simulink model "IDCS_nonlinear"  (R2018a)
settings: Solver=ode4  StartTime=0.0  StopTime=t_end  FixedStep=Step_Time  RelTol=1e-3
values from neighbouring files (symbols this model uses):
  A = [ 0 0 1 0 ... (first row only)    [bode_IDCS.m]    (also in bode_hiratsuka_IDCS.m = 1; hiratsuka_IDCS.m = 0.003; model_IDCS.m = 0.003; model_hiratsuka_nondamper.m = 0.003)
  Aor = 0.1*10^-6    (= 1e-07)    [bode_hiratsuka_IDCS.m]    (also in hiratsuka_IDCS.m; model_hiratsuka_nondamper.m; model_nonlinear_damper.m; model_nonlinear_nondamper.m)
  Ap = (32.50*0.001)^2*pi/4    (= 0.000829576810089)    [bode_hiratsuka_IDCS.m]    (also in hiratsuka_IDCS.m; model_hiratsuka_nondamper.m; model_nonlinear_damper.m; model_nonlinear_nondamper.m)
  B = [0; 0; k1/m1; 0]    [bode_IDCS.m]    (also in bode_hiratsuka_IDCS.m = 0; hiratsuka_IDCS.m = 0; model_hiratsuka_nondamper.m = 0; model_nonlinear_damper.m = 0)
  c1 = 150    [bode_hiratsuka_IDCS.m]    (also in hiratsuka_IDCS.m = 5; model_IDCS.m = 5; model_hiratsuka_nondamper.m = 15; model_linear_damper.m = 50)
  c2 = 7    [bode_IDCS.m]    (also in bode_hiratsuka_IDCS.m; hiratsuka_IDCS.m; model_IDCS.m; model_hiratsuka_nondamper.m)
  Cor = 0.8    [bode_hiratsuka_IDCS.m]    (also in hiratsuka_IDCS.m; model_hiratsuka_nondamper.m; model_nonlinear_damper.m; model_nonlinear_nondamper.m)
  Hz = wv(k)    [bode_hiratsuka_IDCS.m]    (also in hiratsuka_IDCS.m = 6.28318530718; model_IDCS.m = 6.28318530718; model_hiratsuka_nondamper.m = 6.28318530718; model_linear_damper.m = 18.8495559215)
  k1 = 2200    [bode_IDCS.m]    (also in bode_hiratsuka_IDCS.m; hiratsuka_IDCS.m; model_IDCS.m; model_hiratsuka_nondamper.m)
  k2 = 405    [bode_IDCS.m]    (also in bode_hiratsuka_IDCS.m; hiratsuka_IDCS.m; model_IDCS.m; model_hiratsuka_nondamper.m)
  kappa = 1.4    [bode_hiratsuka_IDCS.m]    (also in hiratsuka_IDCS.m; model_hiratsuka_nondamper.m; model_nonlinear_damper.m; model_nonlinear_nondamper.m)
  Kp = 500    [bode_IDCS.m]    (also in bode_hiratsuka_IDCS.m = 80; hiratsuka_IDCS.m = 60; model_IDCS.m = 100; model_hiratsuka_nondamper.m = 80)
  m1 = 1.5    [bode_IDCS.m]    (also in bode_hiratsuka_IDCS.m; hiratsuka_IDCS.m; model_IDCS.m; model_hiratsuka_nondamper.m)
  m2 = 6.4    [bode_IDCS.m]    (also in bode_hiratsuka_IDCS.m; hiratsuka_IDCS.m; model_IDCS.m; model_hiratsuka_nondamper.m)
  P0 = 101325    [bode_hiratsuka_IDCS.m]    (also in hiratsuka_IDCS.m; model_hiratsuka_nondamper.m; model_nonlinear_damper.m; model_nonlinear_nondamper.m)
  row0 = 1.1841    [bode_hiratsuka_IDCS.m]    (also in hiratsuka_IDCS.m; model_hiratsuka_nondamper.m; model_nonlinear_damper.m; model_nonlinear_nondamper.m)
  T_diff = 1/(2*pi*cutoff)    (= 0.00795774715459)    [bode_IDCS.m]    (also in hiratsuka_IDCS.m = 0.00159154943092; model_IDCS.m = 0.00159154943092; model_hiratsuka_nondamper.m = 0.00159154943092; model_linear_damper.m)
  x0 = 0.05    [bode_hiratsuka_IDCS.m]    (also in hiratsuka_IDCS.m = 0.042; model_hiratsuka_nondamper.m; model_nonlinear_damper.m = 0.042; model_nonlinear_nondamper.m = 0.042)
undefined symbols (not defined in the file or in its folder): Kd, Ki
libraries: simulink x1
settings Model: Creator=Natsu Nakagawa  LastModifiedBy=Natsu Nakagawa
settings DataIOCC: ReturnWorkspaceOutputs=on
settings SFSimCC: SimUseLocalCustomCode=on
settings RTWCC: RTWUseLocalCustomCode=on

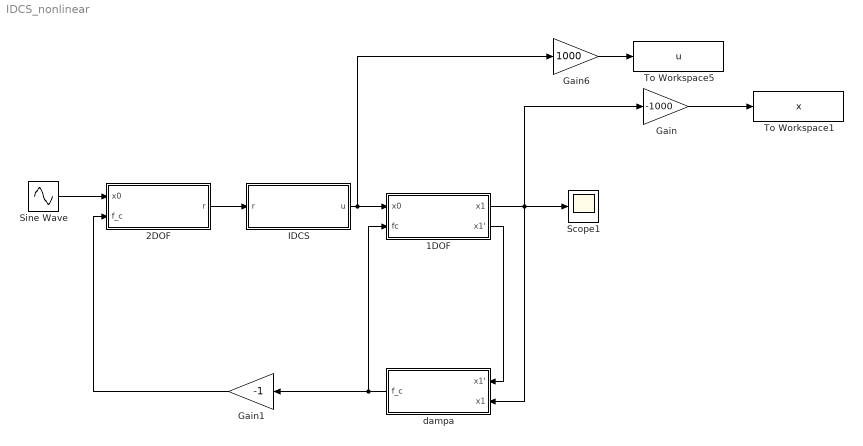
== system IDCS_nonlinear ==
  1DOF : Subsystem
  2DOF : Subsystem
  Gain : Gain  Gain=-1000
  Gain1 : Gain  Gain=-1
  Gain6 : Gain  Gain=1000
  IDCS : Subsystem
  Scope1 : Scope
  Sine Wave : Sin  Amplitude=A  Bias=B  Frequency=Hz  SampleTime=0
  To Workspace1 : ToWorkspace  VariableName=x  SaveFormat=Timeseries  SampleTime=-1
  To Workspace5 : ToWorkspace  VariableName=u  SaveFormat=Timeseries  SampleTime=-1
  dampa : Subsystem
  wires:
  1DOF/1(x1) -> Gain/1, dampa/2(x1), Scope1/1
  2DOF/1(r) -> IDCS/1(r)
  Sine Wave/1 -> 2DOF/1(x0)
  Gain6/1 -> To Workspace5/1
  Gain/1 -> To Workspace1/1
  IDCS/1(u) -> Gain6/1, 1DOF/1(x0)
  1DOF/2(x1') -> dampa/1(x1')
  dampa/1(f_c) -> Gain1/1, 1DOF/2(fc)
  Gain1/1 -> 2DOF/2(f_c)

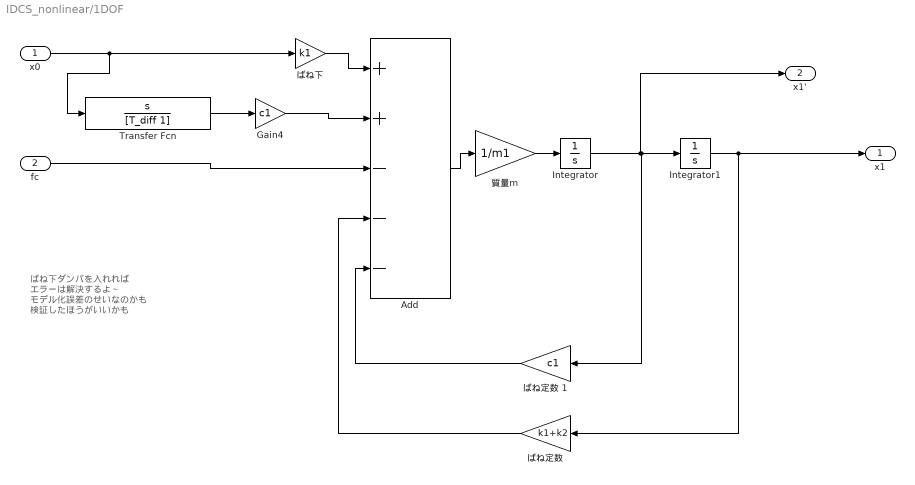
== system IDCS_nonlinear/1DOF ==
  note: ばね下ダンパを入れれば
      | エラーは解決するよ～
      | モデル化誤差のせいなのかも
      | 検証したほうがいいかも
  x0 : Inport
  fc : Inport  Port=2
  Add : Sum  Inputs=++---
  Gain4 : Gain  Gain=c1
  Integrator : Integrator
  Integrator1 : Integrator
  Transfer Fcn : TransferFcn  Numerator=[1, 0]  Denominator=[T_diff 1]
  ばね下 : Gain  Gain=k1
  "ばね定数 " : Gain  Gain=k1+k2
  ばね定数 1 : Gain  Gain=c1
  質量m : Gain  Gain=1/m1
  x1 : Outport
  x1' : Outport  Port=2
  wires:
  Integrator/1 -> x1'/1, ばね定数 1/1, Integrator1/1
  Add/1 -> 質量m/1
  質量m/1 -> Integrator/1
  Integrator1/1 -> x1/1, "ばね定数 "/1
  ばね下/1 -> Add/1
  x0/1 -> Transfer Fcn/1, ばね下/1
  Gain4/1 -> Add/2
  Transfer Fcn/1 -> Gain4/1
  fc/1 -> Add/3
  "ばね定数 "/1 -> Add/4
  ばね定数 1/1 -> Add/5

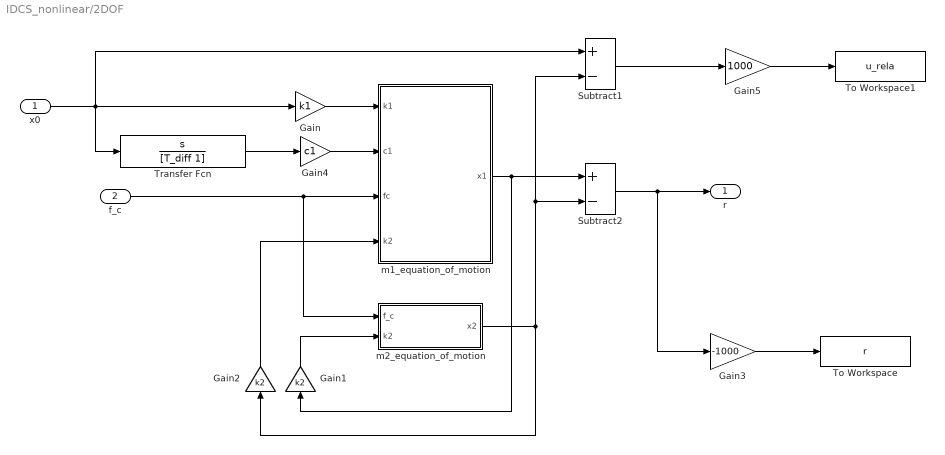
== system IDCS_nonlinear/2DOF ==
  x0 : Inport
  f_c : Inport  Port=2
  Gain : Gain  Gain=k1
  Gain1 : Gain  Gain=k2
  Gain2 : Gain  Gain=k2
  Gain3 : Gain  Gain=-1000
  Gain4 : Gain  Gain=c1
  Gain5 : Gain  Gain=1000
  Subtract1 : Sum  Inputs=+-
  Subtract2 : Sum  Inputs=+-
  To Workspace : ToWorkspace  VariableName=r  SaveFormat=Timeseries  SampleTime=-1
  To Workspace1 : ToWorkspace  VariableName=u_rela  SaveFormat=Timeseries  SampleTime=-1
  Transfer Fcn : TransferFcn  Numerator=[1 0]  Denominator=[T_diff 1]
  m1_equation_of_motion : Subsystem
  m2_equation_of_motion : Subsystem
  r : Outport
  wires:
  x0/1 -> Subtract1/1, Gain/1, Transfer Fcn/1
  Gain/1 -> m1_equation_of_motion/1(k1)
  m1_equation_of_motion/1(x1) -> Subtract2/1, Gain1/1
  f_c/1 -> m2_equation_of_motion/1(f_c), m1_equation_of_motion/3(fc)
  Gain1/1 -> m2_equation_of_motion/2("k2 ")
  Gain3/1 -> To Workspace/1
  m2_equation_of_motion/1(x2) -> Gain2/1, Subtract1/2, Subtract2/2
  Subtract2/1 -> r/1, Gain3/1
  Gain2/1 -> m1_equation_of_motion/4(k2)
  Transfer Fcn/1 -> Gain4/1
  Gain4/1 -> m1_equation_of_motion/2(c1)
  Gain5/1 -> To Workspace1/1
  Subtract1/1 -> Gain5/1

== system IDCS_nonlinear/IDCS ==
  r : Inport
  PID Controller : simulink/Continuous/PID Controller  Controller=P  Form=Ideal  TimeDomain=Continuous-time  SampleTime=-1  IntegratorMethod=Forward Euler  FilterMethod=Forward Euler  ControllerParametersSource=internal  P=Kp  I=Ki  D=Kd  UseFilter=on  N=100  TunerSelectOption=Transfer Function Based (PID Tuner App)  InitialConditionSource=internal  InitialConditionForIntegrator=0  InitialConditionForFilter=0  DifferentiatorICPrevScaledInput=0  ExternalReset=none  TrackingMode=off  Kt=1  LimitOutput=off  UpperSaturationLimit=inf  LowerSaturationLimit=-inf  LinearizeAsGain=on  AntiWindupMode=none  Kb=1  POutMin=[]  POutMax=[]  IOutMin=[]  IOutMax=[]  DOutMin=[]  DOutMax=[]  NOutMin=[]  NOutMax=[]  SumOutMin=[]  SumOutMax=[]  SaturationOutMin=[]  SaturationOutMax=[]  PParamMin=[]  PParamMax=[]  IParamMin=[]  IParamMax=[]  DParamMin=[]  DParamMax=[]  NParamMin=[]  NParamMax=[]  KbParamMin=[]  KbParamMax=[]  KtParamMin=[]  KtParamMax=[]  KbOutMin=[]  KbOutMax=[]  KtOutMin=[]  KtOutMax=[]  IntegratorOutMin=[]  IntegratorOutMax=[]  FilterOutMin=[]  FilterOutMax=[]  SumI1OutMin=[]  SumI1OutMax=[]  SumI2OutMin=[]  SumI2OutMax=[]  SumI3OutMin=[]  SumI3OutMax=[]  SumDOutMin=[]  SumDOutMax=[]  DifferentiatorOutMin=[]  DifferentiatorOutMax=[]  FilterDiffOutCoefMin=[]  FilterDiffOutCoefMax=[]  ReciprocalOutMin=[]  ReciprocalOutMax=[]  SumDenOutMin=[]  SumDenOutMax=[]  SumNumOutMin=[]  SumNumOutMax=[]  DivideOutMin=[]  DivideOutMax=[]  IntegratorContinuousStateAttributes=''  IntegratorStateMustResolveToSignalObject=off  IntegratorRTWStateStorageClass=Auto  FilterContinuousStateAttributes=''  FilterStateMustResolveToSignalObject=off  FilterRTWStateStorageClass=Auto
  Pm : Subsystem
  Sum : Sum  Inputs=|+-
  dampa : Subsystem
  u : Outport
  wires:
  r/1 -> Sum/1
  Sum/1 -> PID Controller/1
  PID Controller/1 -> u/1, Pm/1(x0)
  Pm/1(x1) -> dampa/2(x1), Sum/2
  Pm/2(x1') -> dampa/1(x1')
  dampa/1(f_c) -> Pm/2(fc)

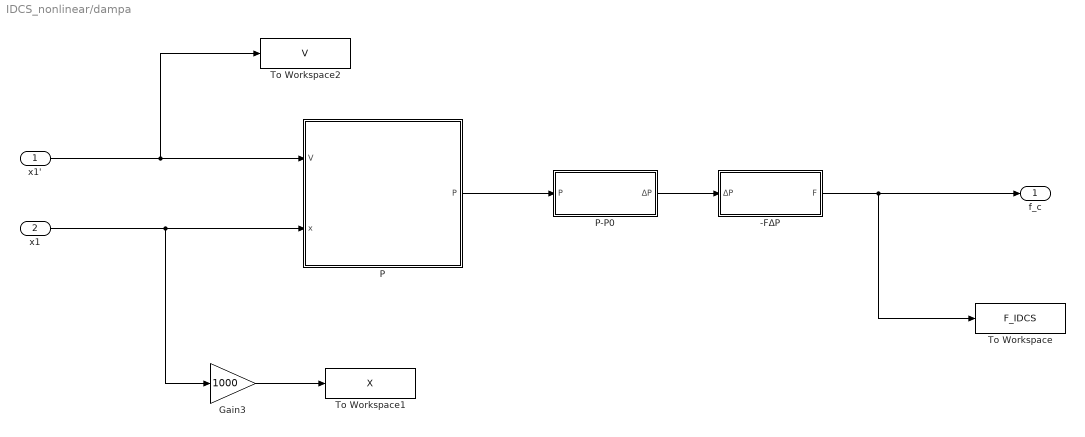
== system IDCS_nonlinear/dampa ==
  x1' : Inport
  x1 : Inport  Port=2
  -FΔP : Subsystem
  Gain3 : Gain  Gain=1000
  P : Subsystem
  P-P0 : Subsystem
  To Workspace : ToWorkspace  VariableName=F_IDCS  SaveFormat=Timeseries  SampleTime=-1
  To Workspace1 : ToWorkspace  VariableName=X  SaveFormat=Timeseries  SampleTime=-1
  To Workspace2 : ToWorkspace  VariableName=V  SaveFormat=Timeseries  SampleTime=-1
  f_c : Outport
  wires:
  x1'/1 -> To Workspace2/1, P/1(V)
  P/1(P) -> P-P0/1(P)
  P-P0/1(ΔP) -> -FΔP/1(ΔP)
  x1/1 -> Gain3/1, P/2(x)
  -FΔP/1(F) -> To Workspace/1, f_c/1
  Gain3/1 -> To Workspace1/1

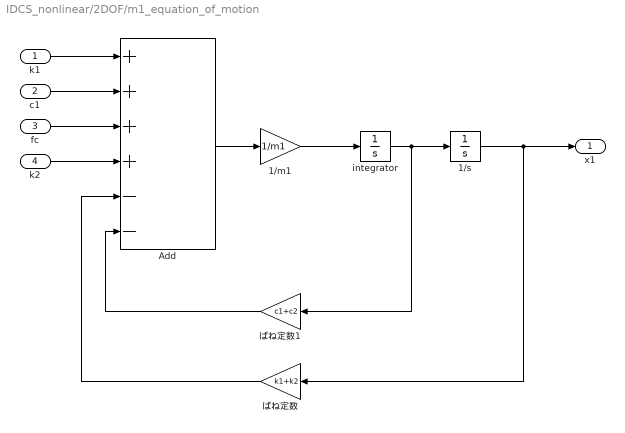
== system IDCS_nonlinear/2DOF/m1_equation_of_motion ==
  k1 : Inport
  c1 : Inport  Port=2
  fc : Inport  Port=3
  k2 : Inport  Port=4
  1/m1 : Gain  Gain=1/m1
  1/s : Integrator
  Add : Sum  Inputs=++++--
  integrator : Integrator
  ばね定数 : Gain  Gain=k1+k2
  ばね定数1 : Gain  Gain=c1+c2
  x1 : Outport
  wires:
  k1/1 -> Add/1
  Add/1 -> 1/m1/1
  integrator/1 -> ばね定数1/1, 1/s/1
  1/s/1 -> x1/1, ばね定数/1
  1/m1/1 -> integrator/1
  ばね定数1/1 -> Add/6
  ばね定数/1 -> Add/5
  fc/1 -> Add/3
  c1/1 -> Add/2
  k2/1 -> Add/4

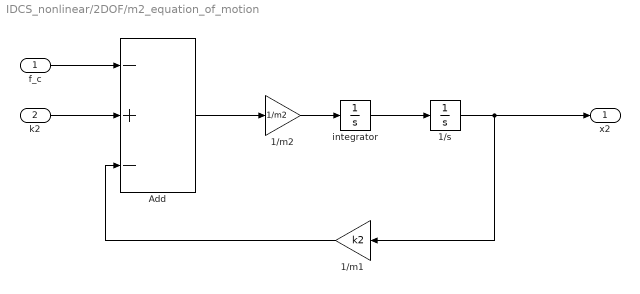
== system IDCS_nonlinear/2DOF/m2_equation_of_motion ==
  f_c : Inport
  "k2 " : Inport  Port=2
  1/m1 : Gain  Gain=k2
  1/m2 : Gain  Gain=1/m2
  1/s : Integrator
  Add : Sum  Inputs=-+-
  integrator : Integrator
  x2 : Outport
  wires:
  f_c/1 -> Add/1
  "k2 "/1 -> Add/2
  Add/1 -> 1/m2/1
  integrator/1 -> 1/s/1
  1/s/1 -> 1/m1/1, x2/1
  1/m1/1 -> Add/3
  1/m2/1 -> integrator/1

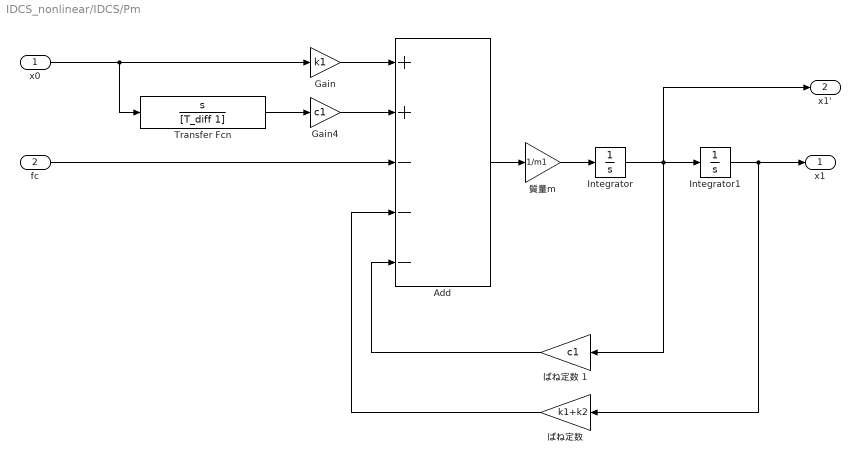
== system IDCS_nonlinear/IDCS/Pm ==
  x0 : Inport
  fc : Inport  Port=2
  Add : Sum  Inputs=++---
  Gain : Gain  Gain=k1
  Gain4 : Gain  Gain=c1
  Integrator : Integrator
  Integrator1 : Integrator
  Transfer Fcn : TransferFcn  Numerator=[1, 0]  Denominator=[T_diff 1]
  "ばね定数 " : Gain  Gain=k1+k2
  ばね定数 1 : Gain  Gain=c1
  質量m : Gain  Gain=1/m1
  x1 : Outport
  x1' : Outport  Port=2
  wires:
  Integrator/1 -> ばね定数 1/1, Integrator1/1, x1'/1
  Add/1 -> 質量m/1
  x0/1 -> Gain/1, Transfer Fcn/1
  質量m/1 -> Integrator/1
  Integrator1/1 -> x1/1, "ばね定数 "/1
  Gain/1 -> Add/1
  fc/1 -> Add/3
  Transfer Fcn/1 -> Gain4/1
  Gain4/1 -> Add/2
  "ばね定数 "/1 -> Add/4
  ばね定数 1/1 -> Add/5

== system IDCS_nonlinear/IDCS/dampa ==
  x1' : Inport
  x1 : Inport  Port=2
  -FΔP : Subsystem
  P : Subsystem
  P-P0 : Subsystem
  f_c : Outport
  wires:
  x1'/1 -> P/1(V)
  P/1(P) -> P-P0/1(P)
  P-P0/1(ΔP) -> -FΔP/1(ΔP)
  x1/1 -> P/2(x)
  -FΔP/1(F) -> f_c/1

== system IDCS_nonlinear/dampa/-FΔP ==
  ΔP : Inport
  Constant : Constant  Value=Ap
  Product : Product
  F : Outport
  wires:
  Constant/1 -> Product/2
  ΔP/1 -> Product/1
  Product/1 -> F/1

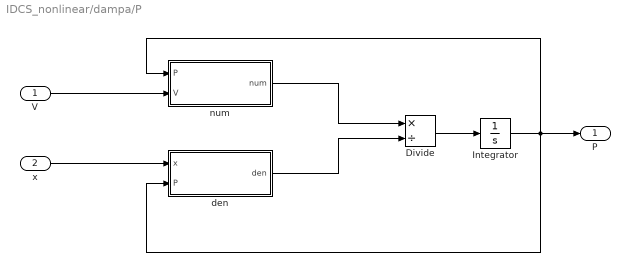
== system IDCS_nonlinear/dampa/P ==
  V : Inport
  x : Inport  Port=2
  Divide : Product  Inputs=*/
  Integrator : Integrator  InitialCondition=P0
  den : Subsystem
  num : Subsystem
  P : Outport
  wires:
  Integrator/1 -> P/1, num/1(P), den/2(P)
  V/1 -> num/2(V)
  Divide/1 -> Integrator/1
  x/1 -> den/1(x)
  den/1(den) -> Divide/2
  num/1(num) -> Divide/1

== system IDCS_nonlinear/dampa/P-P0 ==
  P : Inport
  Add : Sum  Inputs=+-
  Constant : Constant  Value=P0
  ΔP : Outport
  wires:
  P/1 -> Add/1
  Constant/1 -> Add/2
  Add/1 -> ΔP/1

== system IDCS_nonlinear/IDCS/dampa/-FΔP ==
  ΔP : Inport
  Constant : Constant  Value=Ap
  Product : Product
  F : Outport
  wires:
  Constant/1 -> Product/2
  ΔP/1 -> Product/1
  Product/1 -> F/1

== system IDCS_nonlinear/IDCS/dampa/P ==
  V : Inport
  x : Inport  Port=2
  Divide : Product  Inputs=*/
  Integrator : Integrator  InitialCondition=P0
  den : Subsystem
  num : Subsystem
  P : Outport
  wires:
  Integrator/1 -> P/1, num/1(P), den/2(P)
  V/1 -> num/2(V)
  Divide/1 -> Integrator/1
  x/1 -> den/1(x)
  den/1(den) -> Divide/2
  num/1(num) -> Divide/1

== system IDCS_nonlinear/IDCS/dampa/P-P0 ==
  P : Inport
  Add : Sum  Inputs=+-
  Constant : Constant  Value=P0
  ΔP : Outport
  wires:
  P/1 -> Add/1
  Constant/1 -> Add/2
  Add/1 -> ΔP/1

== system IDCS_nonlinear/dampa/P/den ==
  x : Inport
  P : Inport  Port=2
  Product : Product
  Subsystem : Subsystem
  Subsystem1 : Subsystem
  den : Outport
  wires:
  x/1 -> Subsystem/1(x)
  P/1 -> Subsystem1/1(P)
  Subsystem1/1(Out1) -> Product/1
  Subsystem/1(Out1) -> Product/2
  Product/1 -> den/1

== system IDCS_nonlinear/dampa/P/num ==
  P : Inport
  V : Inport  Port=2
  + : Subsystem
  - : Subsystem
  Subtract : Sum  Inputs=-+
  num : Outport
  wires:
  V/1 -> +/2(V)
  P/1 -> -/1(P), +/1(P)
  +/1(Out1) -> Subtract/2
  -/1(Out1) -> Subtract/1
  Subtract/1 -> num/1

== system IDCS_nonlinear/IDCS/dampa/P/den ==
  x : Inport
  P : Inport  Port=2
  Product : Product
  Subsystem : Subsystem
  Subsystem1 : Subsystem
  den : Outport
  wires:
  x/1 -> Subsystem/1(x)
  P/1 -> Subsystem1/1(P)
  Subsystem1/1(Out1) -> Product/1
  Subsystem/1(Out1) -> Product/2
  Product/1 -> den/1

== system IDCS_nonlinear/IDCS/dampa/P/num ==
  P : Inport
  V : Inport  Port=2
  + : Subsystem
  - : Subsystem
  Subtract : Sum  Inputs=-+
  num : Outport
  wires:
  V/1 -> +/2(V)
  P/1 -> -/1(P), +/1(P)
  +/1(Out1) -> Subtract/2
  -/1(Out1) -> Subtract/1
  Subtract/1 -> num/1

== system IDCS_nonlinear/dampa/P/den/Subsystem ==
  x : Inport
  Add : Sum  Inputs=+-
  Constant1 : Constant
  Gain : Gain  Gain=1/x0
  Out1 : Outport
  wires:
  Gain/1 -> Add/2
  Constant1/1 -> Add/1
  Add/1 -> Out1/1
  x/1 -> Gain/1

== system IDCS_nonlinear/dampa/P/den/Subsystem1 ==
  P : Inport
  Constant : Constant  Value=(1/kappa)-1
  Gain : Gain  Gain=1/P0
  Gain1 : Gain  Gain=1/(kappa*P0)
  Pow1 : Math  Operator=pow  OutputSignalType=real  SaturateOnIntegerOverflow=on
  Out1 : Outport
  wires:
  P/1 -> Gain/1
  Gain/1 -> Pow1/1
  Constant/1 -> Pow1/2
  Gain1/1 -> Out1/1
  Pow1/1 -> Gain1/1

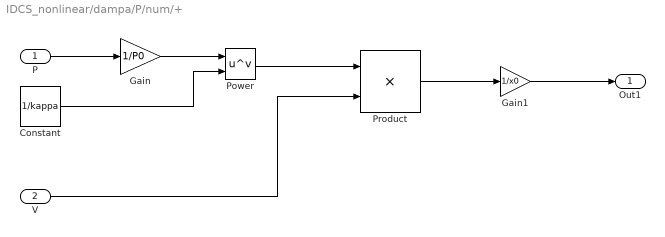
== system IDCS_nonlinear/dampa/P/num/+ ==
  P : Inport
  V : Inport  Port=2
  Constant : Constant  Value=1/kappa
  Gain : Gain  Gain=1/P0
  Gain1 : Gain  Gain=1/x0
  Power : Math  Operator=pow  OutputSignalType=real  SaturateOnIntegerOverflow=on
  Product : Product
  Out1 : Outport
  wires:
  Gain/1 -> Power/1
  Constant/1 -> Power/2
  Power/1 -> Product/1
  V/1 -> Product/2
  Gain1/1 -> Out1/1
  Product/1 -> Gain1/1
  P/1 -> Gain/1

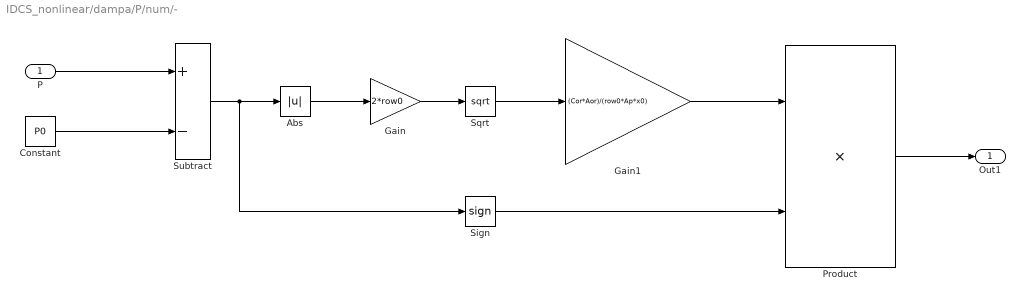
== system IDCS_nonlinear/dampa/P/num/- ==
  P : Inport
  Abs : Abs
  Constant : Constant  Value=P0
  Gain : Gain  Gain=2*row0
  Gain1 : Gain  Gain=(Cor*Aor)/(row0*Ap*x0)
  Product : Product
  Sign : Signum
  Sqrt : Sqrt  SaturateOnIntegerOverflow=on
  Subtract : Sum  Inputs=+-
  Out1 : Outport
  wires:
  Abs/1 -> Gain/1
  Gain/1 -> Sqrt/1
  Sqrt/1 -> Gain1/1
  Sign/1 -> Product/2
  Gain1/1 -> Product/1
  Product/1 -> Out1/1
  Subtract/1 -> Sign/1, Abs/1
  P/1 -> Subtract/1
  Constant/1 -> Subtract/2

== system IDCS_nonlinear/IDCS/dampa/P/den/Subsystem ==
  x : Inport
  Add : Sum  Inputs=+-
  Constant1 : Constant
  Gain : Gain  Gain=1/x0
  Out1 : Outport
  wires:
  Gain/1 -> Add/2
  Constant1/1 -> Add/1
  Add/1 -> Out1/1
  x/1 -> Gain/1

== system IDCS_nonlinear/IDCS/dampa/P/den/Subsystem1 ==
  P : Inport
  Constant : Constant  Value=(1/kappa)-1
  Gain : Gain  Gain=1/P0
  Gain1 : Gain  Gain=1/(kappa*P0)
  Pow1 : Math  Operator=pow  OutputSignalType=real  SaturateOnIntegerOverflow=on
  Out1 : Outport
  wires:
  P/1 -> Gain/1
  Gain/1 -> Pow1/1
  Constant/1 -> Pow1/2
  Gain1/1 -> Out1/1
  Pow1/1 -> Gain1/1

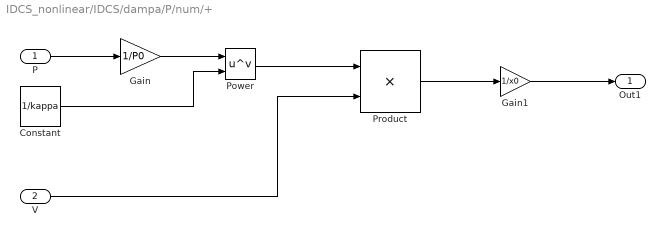
== system IDCS_nonlinear/IDCS/dampa/P/num/+ ==
  P : Inport
  V : Inport  Port=2
  Constant : Constant  Value=1/kappa
  Gain : Gain  Gain=1/P0
  Gain1 : Gain  Gain=1/x0
  Power : Math  Operator=pow  OutputSignalType=real  SaturateOnIntegerOverflow=on
  Product : Product
  Out1 : Outport
  wires:
  Gain/1 -> Power/1
  Constant/1 -> Power/2
  Power/1 -> Product/1
  V/1 -> Product/2
  Gain1/1 -> Out1/1
  Product/1 -> Gain1/1
  P/1 -> Gain/1

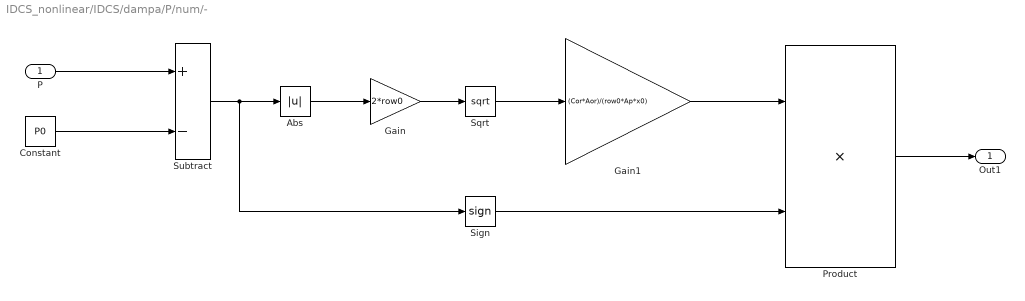
== system IDCS_nonlinear/IDCS/dampa/P/num/- ==
  P : Inport
  Abs : Abs
  Constant : Constant  Value=P0
  Gain : Gain  Gain=2*row0
  Gain1 : Gain  Gain=(Cor*Aor)/(row0*Ap*x0)
  Product : Product
  Sign : Signum
  Sqrt : Sqrt  SaturateOnIntegerOverflow=on
  Subtract : Sum  Inputs=+-
  Out1 : Outport
  wires:
  Abs/1 -> Gain/1
  Gain/1 -> Sqrt/1
  Sqrt/1 -> Gain1/1
  Sign/1 -> Product/2
  Gain1/1 -> Product/1
  Product/1 -> Out1/1
  Subtract/1 -> Sign/1, Abs/1
  P/1 -> Subtract/1
  Constant/1 -> Subtract/2
